simulink model "TentativoPlant"  (R2021a)
settings: Solver=VariableStepAuto  StartTime=0.0  StopTime=10.0  RelTol=1e-3
settings Model: Creator=atavo  LastModifiedBy=atavo

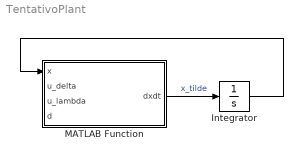
== system TentativoPlant ==
  Integrator : Integrator
  MATLAB Function : MATLAB Function  TreatAsAtomicUnit=on
  wires:
  MATLAB Function/1(dxdt) -> Integrator/1  "x_tilde"
  Integrator/1 -> MATLAB Function/1(x)

== matlab function TentativoPlant/MATLAB Function ==
  data: x input; dxdt output; u_delta input; u_lambda input; d input
function dxdt = Plant(x,u_delta,u_lambda,d)

delta = 0*[1 1 0 0]/180*pi; % 3.5 // 10
delta_rear = ;

rx = [rxf rxf rxr rxr];
ry = [ryf -ryf -ryf ryf];
H = [ones(1,4);
    ry;
    -rx];

x0 = 0;
y0 = 0;
v0 = 130/3.6; % [m/s] vehicle speed
beta0 = 0;
w0 = 0;
psi0 = 0/180*pi;
theta = 15/180*pi;

pinvH = pinv(H);
FzW = pinvH*(rz/2*rho*S*v0^2*[0; Cyb*sin(beta0); -Cx0*cos(beta0)]+[m*g*cos(theta); -rz*m*v0*w0*cos(beta0); -rz*m*g*sin(theta)-rz*m*v0*w0*sin(beta0)]); % forza ground su routa

lambda0s = fsolve(@long_eq,0);
lambda0 = [lambda0s; lambda0s; 0; 0];

Cf = (FzW(1)+FzW(2))*Partial_mu_long(1,0); %cornering stiffness front     partial_mu_long derivata parziale rispetto a beta
Cr = (FzW(3)+FzW(4))*Partial_mu_long(1,0); % rear
A11 = -(Cf+Cr)/(m*v0);
A12 = -v0-(Cf*rxf+Cr*rxr)/(m*v0);
A21 = -(Cf*rxf+Cr*rxr)/(Iz*v0);
A22 = -(Cf*rxf^2+Cr*rxr^2)/(Iz*v0);

A = [A11 A12
     A21 A22];
B1_delta = Cf*[1/m;
    rxf/Iz];

% Quella che aveva fatto lui
B2 = ryf/Iz*[zeros(1,4) ;
    FzW.*[-Partial_mu_long(1,lambda0s) Partial_mu_long(1,lambda0s) Partial_mu_long(1,0) -Partial_mu_long(1,0)]];

% La nostra meno i Lambda che moltiplicano
B1_LAMBDA = [1/m 1/Iz]*[zeros(1,4) Cr;
     [FzW(1)*-Partial_mu_long(1,lambda0s)*ryf FzW(2)*Partial_mu_long(1,lambda0s)*ryf FzW(3)*Partial_mu_long(1,0)*ryf -FzW(4)*Partial_mu_long(1,0)*ryf Cr*rxr]]*[lambda0; delta_rear]; %la matrice funziona mancano i lambda ruote


B2eq = [0; 1/Iz];

C1 = [0 1]; % [-] measured output

y0 = w0; % [rad/s] linearisation output

s = (Cf*rxf+Cr*rxr)/(Cf+Cr);

dxdt = A*x + B1_delta*u_delta + B1_LAMBDA*u_lambda + B2eq*d;
